simulink model "RefModel_SimpleUavMotion"  (R2020a)
settings: Solver=ode1  StartTime=0.0  StopTime=10.0  FixedStep=Ts_Task.Ts_base  RelTol=1e-3
undefined symbols (not defined in the file or in its folder): alt, DiscIntNeverNeededParam, ENUM_FlightControlMode, ENUM_UAVMode, eulerd_yaw_pitch_roll, initialAlignmentCompleteFlag, isHeadingRotateFlag, isNavFilterGood, latd, lla, lond, pitchd, posNED, refloc, rolld, TASK_SET, Ts_SimpleUavMotion, velNED, yawd
libraries: simulink x16, discretizedSecondOrderIntegrator x3, discretizing x2
(part 2 of 2)

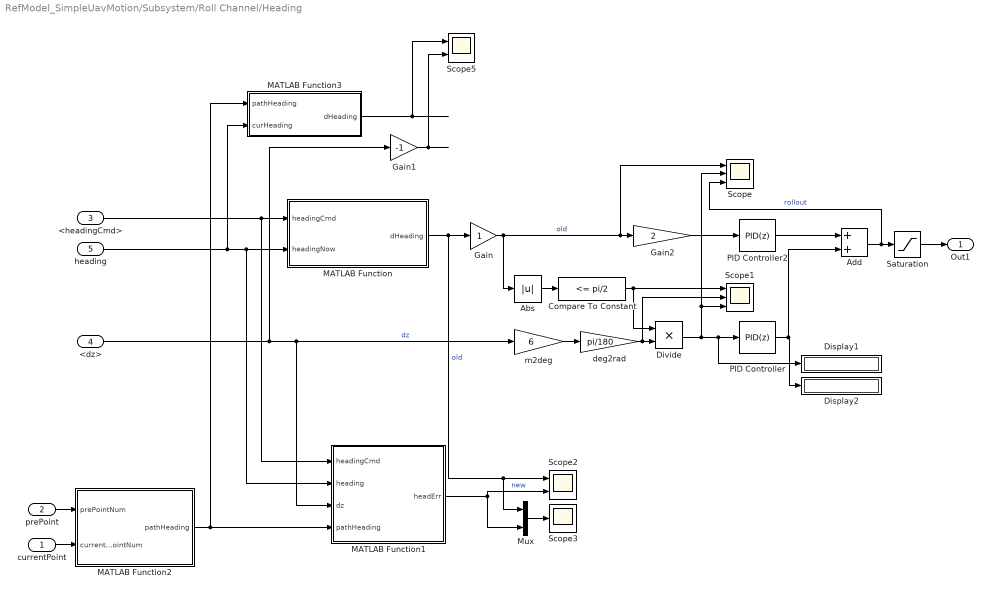
== system RefModel_SimpleUavMotion/Subsystem/Roll Channel/Heading ==
  currentPoint : Inport
  prePoint : Inport  Port=2
  <headingCmd> : Inport  Port=3
  <dz> : Inport  Port=4
  heading : Inport  Port=5
  Abs : Abs
  Add : Sum
  Compare To Constant : simulink/Logic and Bit Operations/Compare To Constant  relop=<=  const=pi/2  OutDataTypeStr=boolean
  Display1 : Display
  Display2 : Display
  Divide : Product  Inputs=**
  Gain : Gain
  Gain1 : Gain  Gain=-1
  Gain2 : Gain  Gain=2
  MATLAB Function : MATLAB Function  TreatAsAtomicUnit=on
  MATLAB Function1 : MATLAB Function  TreatAsAtomicUnit=on
  MATLAB Function2 : MATLAB Function  TreatAsAtomicUnit=on
  MATLAB Function3 : MATLAB Function  TreatAsAtomicUnit=on
  Mux : Mux  Inputs=2
  PID Controller : simulink/Continuous/PID Controller  Controller=PID  Form=Parallel  TimeDomain=Discrete-time  UseExternalTs=off  SampleTime=Ts_SimpleUavMotion.Ts_base  IntegratorMethod=Forward Euler  FilterMethod=Forward Euler  ControllerParametersSource=internal  P=1  I=0  D=2  UseFilter=on  N=24.542109027781645  TunerSelectOption=Transfer Function Based (PID Tuner App)  InitialConditionSource=internal  InitialConditionForIntegrator=0  InitialConditionForFilter=0  DifferentiatorICPrevScaledInput=0  ExternalReset=none  TrackingMode=off  Kt=1  LimitOutput=off  UpperSaturationLimit=50*pi/180  LowerSaturationLimit=-50*pi/180  LinearizeAsGain=on  AntiWindupMode=none  Kb=1  POutMin=[]  POutMax=[]  IOutMin=[]  IOutMax=[]  DOutMin=[]  DOutMax=[]  NOutMin=[]  NOutMax=[]  SumOutMin=[]  SumOutMax=[]  SaturationOutMin=[]  SaturationOutMax=[]  PParamMin=[]  PParamMax=[]  IParamMin=[]  IParamMax=[]  DParamMin=[]  DParamMax=[]  NParamMin=[]  NParamMax=[]  KbParamMin=[]  KbParamMax=[]  KtParamMin=[]  KtParamMax=[]  KbOutMin=[]  KbOutMax=[]  KtOutMin=[]  KtOutMax=[]  IntegratorOutMin=[]  IntegratorOutMax=[]  FilterOutMin=[]  FilterOutMax=[]  SumI1OutMin=[]  SumI1OutMax=[]  SumI2OutMin=[]  SumI2OutMax=[]  SumI3OutMin=[]  SumI3OutMax=[]  SumI4OutMin=[]  SumI4OutMax=[]  SumDOutMin=[]  SumDOutMax=[]  DifferentiatorOutMin=[]  DifferentiatorOutMax=[]  FilterDiffOutCoefMin=[]  FilterDiffOutCoefMax=[]  ReciprocalOutMin=[]  ReciprocalOutMax=[]  SumDenOutMin=[]  SumDenOutMax=[]  SumNumOutMin=[]  SumNumOutMax=[]  DivideOutMin=[]  DivideOutMax=[]  UdiffTsProdOutMin=[]  UdiffTsProdOutMax=[]  NTsProdOutMin=[]  NTsProdOutMax=[]  UintegralTsProdOutMin=[]  UintegralTsProdOutMax=[]  UngainTsProdOutMin=[]  UngainTsProdOutMax=[]  IntegratorContinuousStateAttributes=''  IntegratorStateMustResolveToSignalObject=off  IntegratorRTWStateStorageClass=Auto  FilterContinuousStateAttributes=''  FilterStateMustResolveToSignalObject=off  FilterRTWStateStorageClass=Auto  ParallelPVariant=InternalParameters  IdealPVariant=Disabled  IVariant=InternalParameters  DVariant=InternalParameters  IntegratorVariant=Discrete  SatVariant=Disabled  AWVariant=Passthrough  PCopyVariant=Disabled  TRVariant=Disabled  FdbkBlocksVariant=Forward  IdealPFdbkVariant=Disabled  SatFdbkVariant=Disabled  DerivativeFilterVariant=ForwardEulerFilter  NVariant=InternalParameters  NCopyVariant=Disabled  FilterICVariant=InternalICsFilter  IntegratorICVariant=InternalICs  ExternalResetVariant=Disabled  TRSumVariant=Passthrough  SumFdbkVariant=Disabled  SumVariant=Sum_PID  TsampFilterVariant=InternalTs  TsampNgainVariant=Passthrough  TsampIntegralVariant=Passthrough
  PID Controller2 : simulink/Continuous/PID Controller  Controller=PID  Form=Parallel  TimeDomain=Discrete-time  UseExternalTs=off  SampleTime=Ts_SimpleUavMotion.Ts_base  IntegratorMethod=Forward Euler  FilterMethod=Forward Euler  ControllerParametersSource=internal  P=1.000000000000000  I=0  D=0.000000000000000  UseFilter=on  N=24.542109027781645  TunerSelectOption=Transfer Function Based (PID Tuner App)  InitialConditionSource=internal  InitialConditionForIntegrator=0  InitialConditionForFilter=0  DifferentiatorICPrevScaledInput=0  ExternalReset=none  TrackingMode=off  Kt=1  LimitOutput=off  UpperSaturationLimit=50*pi/180  LowerSaturationLimit=-50*pi/180  LinearizeAsGain=on  AntiWindupMode=none  Kb=1  POutMin=[]  POutMax=[]  IOutMin=[]  IOutMax=[]  DOutMin=[]  DOutMax=[]  NOutMin=[]  NOutMax=[]  SumOutMin=[]  SumOutMax=[]  SaturationOutMin=[]  SaturationOutMax=[]  PParamMin=[]  PParamMax=[]  IParamMin=[]  IParamMax=[]  DParamMin=[]  DParamMax=[]  NParamMin=[]  NParamMax=[]  KbParamMin=[]  KbParamMax=[]  KtParamMin=[]  KtParamMax=[]  KbOutMin=[]  KbOutMax=[]  KtOutMin=[]  KtOutMax=[]  IntegratorOutMin=[]  IntegratorOutMax=[]  FilterOutMin=[]  FilterOutMax=[]  SumI1OutMin=[]  SumI1OutMax=[]  SumI2OutMin=[]  SumI2OutMax=[]  SumI3OutMin=[]  SumI3OutMax=[]  SumI4OutMin=[]  SumI4OutMax=[]  SumDOutMin=[]  SumDOutMax=[]  DifferentiatorOutMin=[]  DifferentiatorOutMax=[]  FilterDiffOutCoefMin=[]  FilterDiffOutCoefMax=[]  ReciprocalOutMin=[]  ReciprocalOutMax=[]  SumDenOutMin=[]  SumDenOutMax=[]  SumNumOutMin=[]  SumNumOutMax=[]  DivideOutMin=[]  DivideOutMax=[]  UdiffTsProdOutMin=[]  UdiffTsProdOutMax=[]  NTsProdOutMin=[]  NTsProdOutMax=[]  UintegralTsProdOutMin=[]  UintegralTsProdOutMax=[]  UngainTsProdOutMin=[]  UngainTsProdOutMax=[]  IntegratorContinuousStateAttributes=''  IntegratorStateMustResolveToSignalObject=off  IntegratorRTWStateStorageClass=Auto  FilterContinuousStateAttributes=''  FilterStateMustResolveToSignalObject=off  FilterRTWStateStorageClass=Auto  ParallelPVariant=InternalParameters  IdealPVariant=Disabled  IVariant=InternalParameters  DVariant=InternalParameters  IntegratorVariant=Discrete  SatVariant=Disabled  AWVariant=Passthrough  PCopyVariant=Disabled  TRVariant=Disabled  FdbkBlocksVariant=Forward  IdealPFdbkVariant=Disabled  SatFdbkVariant=Disabled  DerivativeFilterVariant=ForwardEulerFilter  NVariant=InternalParameters  NCopyVariant=Disabled  FilterICVariant=InternalICsFilter  IntegratorICVariant=InternalICs  ExternalResetVariant=Disabled  TRSumVariant=Passthrough  SumFdbkVariant=Disabled  SumVariant=Sum_PID  TsampFilterVariant=InternalTs  TsampNgainVariant=Passthrough  TsampIntegralVariant=Passthrough
  Saturation : Saturate  UpperLimit=50*pi/180  LowerLimit=-50*pi/180
  Scope : Scope  NumInputPorts=3
  Scope1 : Scope  NumInputPorts=3
  Scope2 : Scope  NumInputPorts=2
  Scope3 : Scope
  Scope5 : Scope  NumInputPorts=2
  deg2rad : Gain  Gain=pi/180
  m2deg : Gain  Gain=6
  Out1 : Outport
  wires:
  <headingCmd>/1 -> MATLAB Function1/1(headingCmd), MATLAB Function/1(headingCmd)
  heading/1 -> MATLAB Function3/2(curHeading), MATLAB Function/2(headingNow), MATLAB Function1/2(heading)
  Gain2/1 -> PID Controller2/1
  <dz>/1 -> Gain1/1, MATLAB Function1/3(dz), m2deg/1  "dz"
  m2deg/1 -> deg2rad/1
  PID Controller/1 -> Add/2, Display2/1
  Divide/1 -> Scope1/3, Scope/2, Display1/1, PID Controller/1
  PID Controller2/1 -> Add/1
  Add/1 -> Scope/3, Saturation/1  "rollout"
  Saturation/1 -> Out1/1
  Abs/1 -> Compare To Constant/1
  Compare To Constant/1 -> Divide/1, Scope1/1
  deg2rad/1 -> Scope1/2, Divide/2
  MATLAB Function1/1(headErr) -> Scope2/2, Mux/2  "new"
  Mux/1 -> Scope3/1
  Gain/1 -> Abs/1, Scope/1, Gain2/1  "old"
  MATLAB Function/1(dHeading) -> Gain/1, Mux/1, Scope2/1  "old"
  Gain1/1 -> Scope5/2
  prePoint/1 -> MATLAB Function2/1(prePointNum)
  currentPoint/1 -> MATLAB Function2/2(currentPointNum)
  MATLAB Function2/1(pathHeading) -> MATLAB Function1/4(pathHeading), MATLAB Function3/1(pathHeading)
  MATLAB Function3/1(dHeading) -> Scope5/1

== system RefModel_SimpleUavMotion/Subsystem/Rotor Height Channel/Height Controller ==
  heightCmd : Inport
  uavMode : Inport  Port=2
  height : Inport  Port=3
  Add : Sum  Inputs=+-
  Atti : Scope  NumInputPorts=4
  Compare To Constant : simulink/Logic and Bit Operations/Compare To Constant  relop===  const=ENUM_UAVMode.Rotor  OutDataTypeStr=boolean
  Divide1 : Product  Inputs=**
  PID Controller2 : simulink/Continuous/PID Controller  Controller=PID  Form=Parallel  TimeDomain=Discrete-time  UseExternalTs=off  SampleTime=Ts_SimpleUavMotion.Ts_base  IntegratorMethod=Forward Euler  FilterMethod=Forward Euler  ControllerParametersSource=internal  P=0.2  I=0  D=0  UseFilter=on  N=50  TunerSelectOption=Transfer Function Based (PID Tuner App)  InitialConditionSource=internal  InitialConditionForIntegrator=0  InitialConditionForFilter=0  DifferentiatorICPrevScaledInput=0  ExternalReset=none  TrackingMode=off  Kt=1  LimitOutput=on  UpperSaturationLimit=2  LowerSaturationLimit=-2  LinearizeAsGain=on  AntiWindupMode=none  Kb=1  POutMin=[]  POutMax=[]  IOutMin=[]  IOutMax=[]  DOutMin=[]  DOutMax=[]  NOutMin=[]  NOutMax=[]  SumOutMin=[]  SumOutMax=[]  SaturationOutMin=[]  SaturationOutMax=[]  PParamMin=[]  PParamMax=[]  IParamMin=[]  IParamMax=[]  DParamMin=[]  DParamMax=[]  NParamMin=[]  NParamMax=[]  KbParamMin=[]  KbParamMax=[]  KtParamMin=[]  KtParamMax=[]  KbOutMin=[]  KbOutMax=[]  KtOutMin=[]  KtOutMax=[]  IntegratorOutMin=[]  IntegratorOutMax=[]  FilterOutMin=[]  FilterOutMax=[]  SumI1OutMin=[]  SumI1OutMax=[]  SumI2OutMin=[]  SumI2OutMax=[]  SumI3OutMin=[]  SumI3OutMax=[]  SumI4OutMin=[]  SumI4OutMax=[]  SumDOutMin=[]  SumDOutMax=[]  DifferentiatorOutMin=[]  DifferentiatorOutMax=[]  FilterDiffOutCoefMin=[]  FilterDiffOutCoefMax=[]  ReciprocalOutMin=[]  ReciprocalOutMax=[]  SumDenOutMin=[]  SumDenOutMax=[]  SumNumOutMin=[]  SumNumOutMax=[]  DivideOutMin=[]  DivideOutMax=[]  UdiffTsProdOutMin=[]  UdiffTsProdOutMax=[]  NTsProdOutMin=[]  NTsProdOutMax=[]  UintegralTsProdOutMin=[]  UintegralTsProdOutMax=[]  UngainTsProdOutMin=[]  UngainTsProdOutMax=[]  IntegratorContinuousStateAttributes=''  IntegratorStateMustResolveToSignalObject=off  IntegratorRTWStateStorageClass=Auto  FilterContinuousStateAttributes=''  FilterStateMustResolveToSignalObject=off  FilterRTWStateStorageClass=Auto  ParallelPVariant=InternalParameters  IdealPVariant=Disabled  IVariant=InternalParameters  DVariant=InternalParameters  IntegratorVariant=Discrete  SatVariant=Enabled  AWVariant=Passthrough  PCopyVariant=Disabled  TRVariant=Disabled  FdbkBlocksVariant=Forward  IdealPFdbkVariant=Disabled  SatFdbkVariant=Disabled  DerivativeFilterVariant=ForwardEulerFilter  NVariant=InternalParameters  NCopyVariant=Disabled  FilterICVariant=InternalICsFilter  IntegratorICVariant=InternalICs  ExternalResetVariant=Disabled  TRSumVariant=Passthrough  SumFdbkVariant=Disabled  SumVariant=Sum_PID  TsampFilterVariant=InternalTs  TsampNgainVariant=Passthrough  TsampIntegralVariant=Passthrough
  heightControl : Outport
  wires:
  Add/1 -> Divide1/2, Atti/4
  Divide1/1 -> PID Controller2/1
  height/1 -> Atti/2, Add/2
  PID Controller2/1 -> heightControl/1, Atti/3
  Compare To Constant/1 -> Divide1/1
  uavMode/1 -> Compare To Constant/1
  heightCmd/1 -> Atti/1, Add/1

== system RefModel_SimpleUavMotion/Subsystem/dHeight/Nonlinear Second-Order Actuator1 ==
  Ac_dem : Inport
  2*zeta * wn : Gain  Gain=2.0 * z_fin* wn_fin  SaturateOnIntegerOverflow=on  OutDataTypeStr=Inherit: Same as input  ParamDataTypeStr=Inherit: Same as input
  Demand limits : Saturate  UpperLimit=fin_max  LowerLimit=fin_min
  "Integrator, Second-Order Limited" : discretizedSecondOrderIntegrator/xLimited  ICSourceX=internal  ICX=fin_act_0  LimitX=on  UpperLimitX=fin_max  LowerLimitX=fin_min  ICSourceDXDT=internal  ICDXDT=fin_act_vel  LimitDXDT=on  UpperLimitDXDT=fin_maxrate  LowerLimitDXDT=-fin_maxrate  ExternalReset=none  IgnoreStateLimitsAndResetForLinearization=off  ReinitDXDTwhenXreachesSaturation=off  ShowOutput=both  GainValue=1.0  SampleTime=Ts_SimpleUavMotion.Ts_base  IntegratorMethod=Integration: Forward Euler
      settings: SourceProductBaseCode=SL
  Sum2 : Sum  Inputs=|+-  InputSameDT=on  SaturateOnIntegerOverflow=on  OutDataTypeStr=Inherit: Same as first input
  Sum3 : Sum  Inputs=|+-  InputSameDT=on  SaturateOnIntegerOverflow=on  OutDataTypeStr=Inherit: Same as first input
  rate limit*2*zeta/wn : Saturate  UpperLimit=fin_maxrate*2*z_fin/wn_fin  LowerLimit=-fin_maxrate*2*z_fin/wn_fin
  wn^2 : Gain  Gain=wn_fin* wn_fin  SaturateOnIntegerOverflow=on  OutDataTypeStr=Inherit: Same as input  ParamDataTypeStr=Inherit: Same as input
  Ac_ac : Outport  InitialOutput=0  VectorParamsAs1DForOutWhenUnconnected=off
  wires:
  "Integrator, Second-Order Limited"/2 -> 2*zeta * wn/1
  "Integrator, Second-Order Limited"/1 -> Ac_ac/1, Sum3/2
  wn^2/1 -> Sum2/1
  Sum2/1 -> "Integrator, Second-Order Limited"/1
  2*zeta * wn/1 -> Sum2/2
  Sum3/1 -> rate limit*2*zeta/wn/1
  rate limit*2*zeta/wn/1 -> wn^2/1
  Demand limits/1 -> Sum3/1
  Ac_dem/1 -> Demand limits/1

== system RefModel_SimpleUavMotion/Subsystem/speed channel/Nonlinear Second-Order Actuator1 ==
  Ac_dem : Inport
  2*zeta * wn : Gain  Gain=2.0 * z_fin* wn_fin  SaturateOnIntegerOverflow=on  OutDataTypeStr=Inherit: Same as input  ParamDataTypeStr=Inherit: Same as input
  Demand limits : Saturate  UpperLimit=fin_max  LowerLimit=fin_min
  "Integrator, Second-Order Limited" : discretizedSecondOrderIntegrator/xLimited  ICSourceX=internal  ICX=fin_act_0  LimitX=on  UpperLimitX=fin_max  LowerLimitX=fin_min  ICSourceDXDT=internal  ICDXDT=fin_act_vel  LimitDXDT=on  UpperLimitDXDT=fin_maxrate  LowerLimitDXDT=-fin_maxrate  ExternalReset=none  IgnoreStateLimitsAndResetForLinearization=off  ReinitDXDTwhenXreachesSaturation=off  ShowOutput=both  GainValue=1.0  SampleTime=Ts_SimpleUavMotion.Ts_base  IntegratorMethod=Integration: Forward Euler
      settings: SourceProductBaseCode=SL
  Sum2 : Sum  Inputs=|+-  InputSameDT=on  SaturateOnIntegerOverflow=on  OutDataTypeStr=Inherit: Same as first input
  Sum3 : Sum  Inputs=|+-  InputSameDT=on  SaturateOnIntegerOverflow=on  OutDataTypeStr=Inherit: Same as first input
  rate limit*2*zeta/wn : Saturate  UpperLimit=fin_maxrate*2*z_fin/wn_fin  LowerLimit=-fin_maxrate*2*z_fin/wn_fin
  wn^2 : Gain  Gain=wn_fin* wn_fin  SaturateOnIntegerOverflow=on  OutDataTypeStr=Inherit: Same as input  ParamDataTypeStr=Inherit: Same as input
  Ac_ac : Outport  InitialOutput=0  VectorParamsAs1DForOutWhenUnconnected=off
  wires:
  Ac_dem/1 -> Demand limits/1
  Demand limits/1 -> Sum3/1
  rate limit*2*zeta/wn/1 -> wn^2/1
  Sum3/1 -> rate limit*2*zeta/wn/1
  2*zeta * wn/1 -> Sum2/2
  Sum2/1 -> "Integrator, Second-Order Limited"/1
  wn^2/1 -> Sum2/1
  "Integrator, Second-Order Limited"/1 -> Sum3/2, Ac_ac/1
  "Integrator, Second-Order Limited"/2 -> 2*zeta * wn/1

== matlab function RefModel_SimpleUavMotion/Subsystem/Roll Channel/Heading/MATLAB Function2 ==
  data: prePointNum input; pathHeading output; currentPointNum input
function pathHeading = fcn(prePointNum, currentPointNum)
prePointNum = reshape(prePointNum,[1,3]);
currentPointNum = reshape(currentPointNum,[1,3]);
curPos = lla2ned(currentPointNum,prePointNum(1:2));
pathHeading = atan2(curPos(2),curPos(1));

== matlab function RefModel_SimpleUavMotion/Subsystem/Heading Dynamics And InnerLoop/HeadingMotion/MATLAB Function2 ==
  data: roll input; dHeading output; speed input
function dHeading = fcn(roll, speed)
if abs(speed) > 0.1
    dHeading = 9.8*tan(roll)/speed;
else
    dHeading = 0;
end

== matlab function RefModel_SimpleUavMotion/Subsystem/speed channel/MATLAB Function ==
  data: autoManualMode input; targetLL input; groundspeed input; curLLA input; velTarget output
function velTarget = fcn(autoManualMode, targetLL, groundspeed, curLLA)
curLL = curLLA(1:2);
dLat = targetLL(1)- curLL(1);
dLon = targetLL(2)- curLL(2);
deg2m = 111e3;
dPn = dLat*deg2m;
dPe = dLon*deg2m*cos(curLL(1)*pi/180);
if autoManualMode ~= ENUM_ControlMode.Manual
    if norm([dPn,dPe]) > 1
        headingTarget = atan2(dPe,dPn);
        velTarget = groundspeed*[cos(headingTarget);sin(headingTarget)];
    else
        velTarget = 0*[1;1];
    end
else
    velTarget = [0;0];
end

== matlab function RefModel_SimpleUavMotion/MATLAB Function1 ==
  data: vn input; speed output; ve input
function speed = fcn(vn, ve)
speed = norm([vn,ve]);

== matlab function RefModel_SimpleUavMotion/Subsystem/Roll Channel/Heading/MATLAB Function3 ==
  data: pathHeading input; dHeading output; curHeading input
function dHeading = fcn(pathHeading,curHeading)
dHeading = angdiff(pathHeading,curHeading);

== stateflow chart RefModel_SimpleUavMotion/BatteryLife Dynamics/BatteryLife_StateFlow ==
  state en_du_
    dot_batterylife = batteryLifeDynamics();
  (default) -> en_du_
  data: y function_output; clock_sec input; taskmode input; uavmode input; dot_batterylife output; FlightPerfParam data_store_memory; curAirSpeed input; curEuler input; curGroundSpeed input; velNED input size=3; windSpeed_ms input; windHeading_rad input
  function y = batteryLifeDynamics:
    | function y = batteryLifeDynamics
    | windSpeedWhenGoHomeAtThisLL = curAirSpeed - curGroundSpeed;
    | cruiseSpeed_cruise = 19;
    | speedmode = 'fixAirspeed';
    | velScale_FixGoHome = 1;
    | switch speedmode
    |     case 'fixAirspeed'
    |         velScale_FixGoHome = cruiseSpeed_cruise / abs( cruiseSpeed_cruise-windSpeedWhenGoHomeAtThisLL);
    |     case 'variableAirspeed'
    |         velScale_FixGoHome = 1 + windSpeedWhenGoHomeAtThisLL/cruiseSpeed_cruise;
    | end
    | 
    | switch taskmode
    |     case ENUM_FlightTaskMode.GroundStandByMode
    |         y = FlightPerfParam.powerRate_GroundStandBy;
    |     case ENUM_FlightTaskMode.TakeOffMode
    |         y = FlightPerfParam.powerRate_RotorUpNoWind;
    |     case ENUM_FlightTaskMode.HoverAdjustMode
    |         y = FlightPerfParam.powerRate_RotorHoverNoWind;
    |     case ENUM_FlightTaskMode.Rotor2Fix_Mode
    |         y = FlightPerfParam.powerRate_RotorHoverNoWind;
    |     case ENUM_FlightTaskMode.Fix2Rotor_Mode
    |         y = FlightPerfParam.powerRate_RotorHoverNoWind;
    |     case ENUM_FlightTaskMode.HoverUpMode
    |         y = FlightPerfParam.powerRate_FixHoverUp;
    |     case ENUM_FlightTaskMode.PathFollowMode
    |         y = velScale_FixGoHome*FlightPerfParam.powerRate_FixCruise;        
    |     case ENUM_FlightTaskMode.GoHomeMode
    |         if uavmode == ENUM_UAVMode.Fix
    |             y = velScale_FixGoHome*FlightPerfParam.powerRate_FixCruise;     
    |         else
    |             y = FlightPerfParam.powerRate_RotorMoveNoWind;     
    |         end
    |     case ENUM_FlightTaskMode.HoverDownMode
    |         y = FlightPerfParam.powerRate_FixHoverDown;  
    |     case ENUM_FlightTaskMode.LandMode
    |         y = FlightPerfParam.powerRate_RotorDownNoWind;       
    |     case ENUM_FlightTaskMode.VerticalMove
    |         Vd = velNED(3);
    |         if Vd > 1
    |             y = FlightPerfParam.powerRate_FixHoverDown;       
    |         elseif Vd < -1
    |             y = FlightPerfParam.powerRate_FixHoverUp;   
    |         else
    |             y = 0;
    |         end
    |     case ENUM_FlightTaskMode.AirStandByMode
    |         y = FlightPerfParam.powerRate_FixHoverLevel;
    |     otherwise
    |         y = 0;
    | end

== matlab function RefModel_SimpleUavMotion/BatteryLife Dynamics/batterySet ==
  data: clock_sec input; mavlink_msg_mission_current input Bus: mavlink_msg_mission_current; mavlink_msg_mission_current output size=3; powerPercent input
function mavlink_msg_mission_current  = fcn(clock_sec,mavlink_msg_mission_current,powerPercent)
for i = 1:3
    if clock_sec < 5
        mavlink_msg_mission_current(i).remaining = int8(0);
        %     mavlink_msg_mission_current(2).remaining = int8(0);
        %     mavlink_msg_mission_current(3).remaining = int8(0);
    else
        mavlink_msg_mission_current(i).remaining = int8(max(0,floor(powerPercent)));
        %     mavlink_msg_mission_current(2).remaining = int8(floor(powerPercent));
        %     mavlink_msg_mission_current(3).remaining = int8(floor(powerPercent));
    end
end

== matlab function RefModel_SimpleUavMotion/Subsystem/MATLAB Function3 ==
  data: dv input; y output
function y = fcn(dv)
persistent meanDv
if isempty(meanDv)
    meanDv = 0; 
end
meanDv = 0.9*meanDv + 0.1*dv;
y = meanDv;

== matlab function RefModel_SimpleUavMotion/Subsystem/MATLAB Function ==
  data: heading input; uavmode input; vn output; speed input; ve output; VnVe_Rotor input
function [vn,ve] = fcn(heading, uavmode, speed, VnVe_Rotor)
if uavmode ~= ENUM_UAVMode.Rotor
    vn = speed*cos(heading);
    ve = speed*sin(heading);
else
    vn = VnVe_Rotor(1);
    ve = VnVe_Rotor(2);
end

== matlab function RefModel_SimpleUavMotion/Subsystem/Roll Dynamics And InnerLoop/MATLAB Function ==
  data: u input; y input
function fcn(u, y)
if isnan(u) || isnan(y)
    sl = 1;
end

== matlab function RefModel_SimpleUavMotion/Subsystem/Roll Channel/Heading/MATLAB Function ==
  data: headingCmd input; dHeading output; headingNow input
function dHeading = calHeadingErr(headingCmd,headingNow)
% 计算飞机当前航向偏差
% headingCmd: 指令航向 rad
% headingNow：当前航向 rad
% dHeading: 航向差 rad
if 0
    headingNow = rem(headingNow,2*pi);
    headingCmd = rem(headingCmd,2*pi);
    sub = zeros(3,1);
    psi_d_possible = zeros(3,1);
    psi_d_possible(1) = headingCmd;
    psi_d_possible(2) = headingCmd-2*pi;
    psi_d_possible(3) = headingCmd+2*pi;
    sub(1) = psi_d_possible(1)-headingNow;
    sub(2) = psi_d_possible(2)-headingNow;
    sub(3) = psi_d_possible(3)-headingNow;
    [~,ind] = min(abs(sub));
    dHeading = sub(ind);
else
    dHeading = -angdiff(headingCmd,headingNow);
end
% dHeading,dHeading1
% sl = 1;

== matlab function RefModel_SimpleUavMotion/MATLAB Function ==
  settings: updateMethod=DISCRETE
  data: lla_out output; vn input; ve input; height_out input; vd input; lla0 input; dt input; velNED_out output; homeLLA input; posNED_out output
function [lla_out,velNED_out,posNED_out] = fcn(vn,ve, height_out, vd, lla0, dt, homeLLA)
persistent lla lla0pre
if isempty(lla)
    lla = lla0;
    lla0pre = lla0;
end
if abs(lla0(1)-lla0pre(1))>1e-5 || abs(lla0(2)-lla0pre(2))>1e-5
    lla = lla0;
    lla0pre = lla0;
end
% vn = speed*cos(heading);
% ve = speed*sin(heading);
lla(1) = lla(1) + 1/111e3*vn*dt;
lla(2) = lla(2) + 1/111e3*ve/cos(lla(1)*pi/180)*dt;
lla(3) = lla0(3) + height_out;
lla_out = lla;
velNED_out = [vn,ve,vd]';
if homeLLA(1) == 0 && homeLLA(2) == 0
    posNED_out = [0,0,0]';
else
    temp = lla2ned(lla_out', homeLLA(1:2));
    posNED_out = temp';
    posNED_out(3) = - posNED_out(3) - homeLLA(3);
end
end

%% 子函数
function p = lla2ned(lla, ll0)
% 纬经高转换为NED位置
% lla: 纬度[deg] 经度[deg] 高度[m]
% ll0: 基准点， 纬度[deg] 经度[deg]
% p: NED位置
p = zeros(1,3);
psi0 = 0;
href = 0;
f = 0.003352810664747;
R = 6378.137e3;
% wrap latitude and longitude if needed
[~, lla(:,1), lla(:,2)] = wraplatitude( lla(:,1), lla(:,2), 'deg' );
[~, ll0(1), ll0(2)] = wraplatitude( ll0(1), ll0(2), 'deg' );

% check and fix angle wrapping in longitude
[~, lla(:,2)] = wraplongitude( lla(:,2), 'deg', '180' );
[~, ll0(2)] = wraplongitude( ll0(2), 'deg', '180' );

dLat = lla(:,1) - ll0(1);
dLon = lla(:,2) - ll0(2);

% wrap latitude and longitude if needed
[~, dLat, dLon] = wraplatitude( dLat', dLon', 'deg' );

% check and fix angle wrapping in longitude
[~, dLon] = wraplongitude( dLon, 'deg', '180' );

rll0 = ll0*pi/180;
rpsi0 = psi0*pi/180;

Rn = R/sqrt(1-(2*f-f*f)*sin(rll0(1))*sin(rll0(1)));
Rm = Rn*((1-(2*f-f*f))/(1-(2*f-f*f)*sin(rll0(1))*sin(rll0(1))));

dNorth = dLat./atan2(1,Rm)*pi/180;
dEast = dLon./atan2(1,Rn*cos(rll0(1)))*pi/180;

p(:,1) = cos(rpsi0)*dNorth + sin(rpsi0)*dEast;
p(:,2) = -sin(rpsi0)*dNorth + cos(rpsi0)*dEast;
p(:,3) = -lla(:,3) - href;
end

function [lat_wrapped, lat, lon] = wraplatitude( lat, lon, units)
% WRAPLATITUDE internal function to check and fix angle wrapping in
% latitude and longitude if needed.

%   Copyright 2007-2013 The MathWorks, Inc.

% Convert units if necessary
if strcmp(units,'deg')
    pideg = 180;
else
    pideg = pi;
end

% Set lat_wrapped flag to false
lat_wrapped = false;

% Re-set latitudes to values between pi and -pi
flat = abs(lat);

if any(flat>pideg)
    lat(flat>pideg) = mod(lat(flat>pideg)+pideg,2*pideg)-pideg;
    % Set lat_wrapped flag to true if necessary
    flat = abs(lat);
    lat_wrapped = true;
end

% Determine if any latitudes need to be wrapped
idx = flat>pideg/2;

if any(idx)
    
    % Adjustments for -pi to pi
    flat = abs(lat);
    latp2 = flat>pideg/2;
    lon(idx) = lon(idx) + pideg;
    lat(latp2) = sign(lat(latp2)).*(pideg/2-(flat(latp2)-pideg/2));
    
    % Set lat_wrapped flag to true if necessary
    lat_wrapped = true;
    
end
end

function [lon_wrapped, lon] = wraplongitude( lon, inputUnits, maxRange )
% WRAPLONGITUDE internal function to check and fix angle wrapping in
% longitude.

%   Copyright 2007-2010 The MathWorks, Inc.

% Convert units if necessary
if strcmp(inputUnits,'deg')
    lon = lon*pi/180;
end

lon_wrapped = false;

switch maxRange
    % Range goes between -pi and pi
    case {'180','pi'}
        idx = lon > pi | lon < -pi;
        if any(idx)
            lon(idx) = rem(lon(idx),2*pi)- (2*pi)*fix(rem(lon(idx),2*pi)/pi);
            lon_wrapped = true;
        end
        % Range goes between 0 and 2*pi
    case {'360','2*pi'}
        idx = lon > 2*pi | lon < 0;
        if any(idx)
            lon(idx) = mod(lon(idx),2*pi);
            lon_wrapped = true;
        end
    otherwise
        % do nothing
end

% Convert units if necessary
if strcmp(inputUnits,'deg')
    lon = lon*180/pi;
end
end

== matlab function RefModel_SimpleUavMotion/Subsystem/Heading Dynamics And InnerLoop/HeadingMotion/-pi,pi ==
  data: u input; y output
function y = fcn(u)
y = rem(u,2*pi);
if y > pi
    y = y-2*pi;
end
if isnan(u) || isnan(y)
    sl = 1;
end

== matlab function RefModel_SimpleUavMotion/Subsystem/Heading Channel/Heading Controller/MATLAB Function1 ==
  data: headingCmd input; dHeading output; headingNow input
function dHeading = calHeadingErr(headingCmd,headingNow)
% 计算飞机当前航向偏差
% headingCmd: 指令航向 rad
% headingNow：当前航向 rad
% dHeading: 航向差 rad
if 0
    headingNow = rem(headingNow,2*pi);
    headingCmd = rem(headingCmd,2*pi);
    sub = zeros(3,1);
    psi_d_possible = zeros(3,1);
    psi_d_possible(1) = headingCmd;
    psi_d_possible(2) = headingCmd-2*pi;
    psi_d_possible(3) = headingCmd+2*pi;
    sub(1) = psi_d_possible(1)-headingNow;
    sub(2) = psi_d_possible(2)-headingNow;
    sub(3) = psi_d_possible(3)-headingNow;
    [~,ind] = min(abs(sub));
    dHeading = sub(ind);
else
    dHeading = -angdiff(headingCmd,headingNow);
end

== matlab function RefModel_SimpleUavMotion/MATLAB Function2 ==
  data: lla0 input; lla0_GroundStationSet input; y output; taskMode input
function y = fcn(lla0, lla0_GroundStationSet, taskMode)
persistent pLLA0
if isempty(pLLA0)
    pLLA0 = [0,0,0]';
end
if taskMode == ENUM_FlightTaskMode.GroundStandByMode || ...
        taskMode == ENUM_FlightTaskMode.NoneFlightTaskMode
    if lla0_GroundStationSet(1) ~= 0 && abs(lla0_GroundStationSet(1)) < 100
        y = lla0_GroundStationSet;
    %     y(3) = 0;
    else
        y = lla0;
    end
    pLLA0 = y;
else
    y = pLLA0;
end

== matlab function RefModel_SimpleUavMotion/Subsystem/Roll Channel/Heading/MATLAB Function1 ==
  data: headingCmd input; headErr output; heading input; dz input; pathHeading input
function headErr = fcn(headingCmd, heading, dz, pathHeading)
if abs(dz) < 5
    k = 0.3;
else
    k = 0.3;
end
angle = abs(dz)*pi/180;
dheading = min(k*angle,60*pi/180);
if dz > 0 % 俯视，uav在航线左侧
    headingCmd = pathHeading + dheading;
elseif dz < 0
    headingCmd = pathHeading - dheading;
else
    headingCmd = headingCmd;
end
headErr = angdiff(heading,headingCmd);
